simulink library "processRawData"  (R2020a)
settings: Solver=VariableStepAuto  StartTime=0.0  StopTime=10.0  RelTol=1e-3
libraries: simulink x1, MovingAverageFilter x1
settings Model: Creator=Ayaz  LastModifiedBy=Ayaz

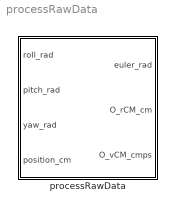
== system processRawData ==
  processRawData : Subsystem  mask{FilterWindowSize=20}
      mask prompts: FilterWindowSize "Filter window size"
      mask TypeOptions FilterWindowSize: Subsystem/moving average filter/FilterWindowSize

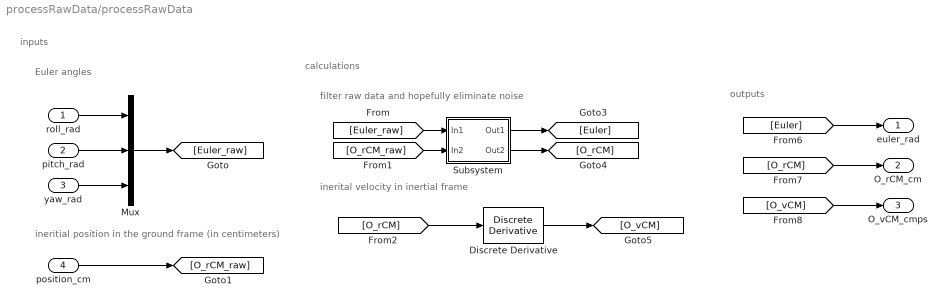
== system processRawData/processRawData ==
  note: outputs
  note: calculations
  note: inerital velocity in inertial frame
  note: filter raw data and hopefully eliminate noise
  note: inputs
  note: ineritial position in the ground frame
      | (in centimeters)
  note: Euler angles
  roll_rad : Inport
  pitch_rad : Inport  Port=2
  yaw_rad : Inport  Port=3
  position_cm : Inport  Port=4
  Discrete Derivative : simulink/Quick Insert/Discrete/Discrete Derivative  gainval=1.0  ICPrevScaledInput=0.0  OutMin=[]  OutMax=[]  OutDataType=fixdt(1, 16)  OutScaling=2^-10  DoSatur=off
      settings: SourceProductBaseCode=SL
  Mux : Mux  Inputs=3
  Subsystem : Subsystem
  euler_rad : Outport
  O_rCM_cm : Outport  Port=2
  O_vCM_cmps : Outport  Port=3
  wires:
  pitch_rad/1 -> Mux/2
  roll_rad/1 -> Mux/1
  yaw_rad/1 -> Mux/3
  Mux/1 -> [Euler_raw]
  position_cm/1 -> [O_rCM_raw]
  [Euler_raw] -> Subsystem/1(In1)
  [O_rCM_raw] -> Subsystem/2(In2)
  Subsystem/1(Out1) -> [Euler]
  Subsystem/2(Out2) -> [O_rCM]
  [O_rCM] -> Discrete Derivative/1
  Discrete Derivative/1 -> [O_vCM]
  [Euler] -> euler_rad/1
  [O_rCM] -> O_rCM_cm/1
  [O_vCM] -> O_vCM_cmps/1

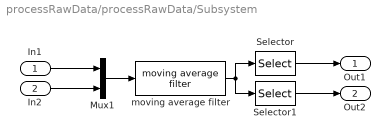
== system processRawData/processRawData/Subsystem ==
  In1 : Inport
  In2 : Inport  Port=2
  Mux1 : Mux  Inputs=2
  Selector : Selector  InputPortWidth=6  IndexOptions=Index vector (dialog)  Indices=[1 2 3]  OutputSizes=1
  Selector1 : Selector  InputPortWidth=6  IndexOptions=Index vector (dialog)  Indices=[4 5 6]  OutputSizes=1
  moving average filter : MovingAverageFilter/moving average filter  FilterWindowSize=FilterWindowSize
  Out1 : Outport
  Out2 : Outport  Port=2
  wires:
  In2/1 -> Mux1/2
  moving average filter/1 -> Selector/1, Selector1/1
  Mux1/1 -> moving average filter/1
  In1/1 -> Mux1/1
  Selector1/1 -> Out2/1
  Selector/1 -> Out1/1
